simulink model "project3_week2"  (R2021a)
settings: Solver=ode45  StartTime=0.0  StopTime=120  RelTol=1e-3
model workspace (MAT data in the model file):
  b = Simulink.Parameter
  b.Value = 50
  b.DataType = 'auto'
  b.Dimensions = [1 1]
  ki = Simulink.Parameter
  ki.Value = 50
  ki.DataType = 'auto'
  ki.Dimensions = [1 1]
  kp = Simulink.Parameter
  kp.Value = 40
  kp.DataType = 'auto'
  kp.Dimensions = [1 1]
  m = Simulink.Parameter
  m.Value = 1000
  m.DataType = 'auto'
  m.Dimensions = [1 1]
  u = Simulink.Parameter
  u.Value = 500
  u.DataType = 'auto'
  u.Dimensions = [1 1]
settings Model: DataDictionary=DATA_cruise_control.sldd  EnableAccessToBaseWorkspace=off  Creator=RASIKA MALGI  LastModifiedBy=RASIKA MALGI
settings SolverCC: AlgebraicLoopSolver=TrustRegion
settings DebuggingCC: SFMachineParentedDataDiag=warning

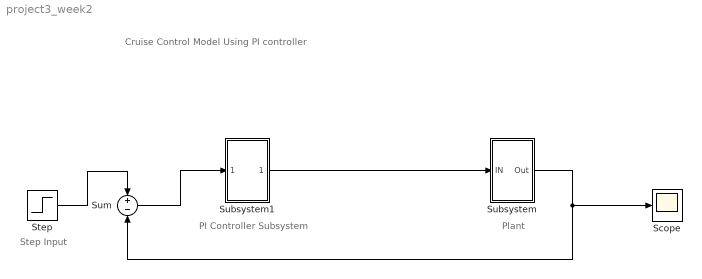
== system project3_week2 ==
  note: Cruise Control Model Using PI controller
  note: Step Input
  note: Plant
  note: PI Controller Subsystem
  Scope : Scope
  Step : Step  Time=0  After=u  SampleTime=0
  Subsystem : Subsystem
  Subsystem1 : Subsystem
  Sum : Sum  Inputs=+-
  wires:
  Subsystem1/1(Out1) -> Subsystem/1(IN)
  Step/1 -> Sum/1
  Sum/1 -> Subsystem1/1(In1)
  Subsystem/1(Out) -> Sum/2, Scope/1

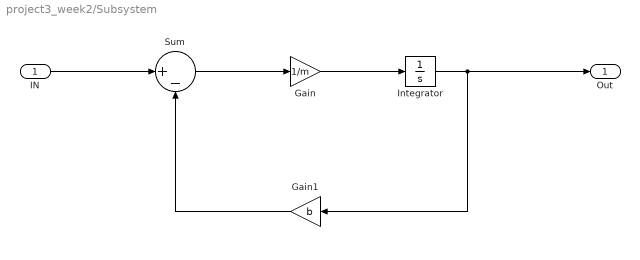
== system project3_week2/Subsystem ==
  IN : Inport
  Gain : Gain  Gain=1/m
  Gain1 : Gain  Gain=b
  Integrator : Integrator
  Sum : Sum  Inputs=|+-
  Out : Outport
  wires:
  Gain/1 -> Integrator/1
  Integrator/1 -> Out/1, Gain1/1
  Sum/1 -> Gain/1
  Gain1/1 -> Sum/2
  IN/1 -> Sum/1

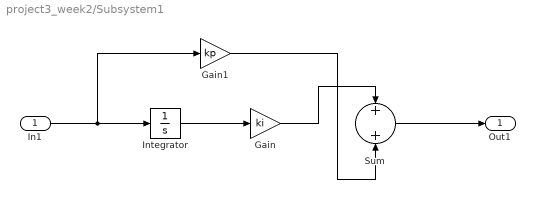
== system project3_week2/Subsystem1 ==
  In1 : Inport
  Gain : Gain  Gain=ki
  Gain1 : Gain  Gain=kp
  Integrator : Integrator
  Sum : Sum
  Out1 : Outport
  wires:
  Integrator/1 -> Gain/1
  Gain1/1 -> Sum/2
  In1/1 -> Gain1/1, Integrator/1
  Sum/1 -> Out1/1
  Gain/1 -> Sum/1
